simulink model "Sim01_BangBang"  (R2021a)
settings: Solver=FixedStepAuto  StartTime=0.0  StopTime=T  FixedStep=Ts  RelTol=1e-3
values from neighbouring files (symbols this model uses):
  Ts = 1e-3    (= 0.001)    [Sim01_Stability.m]    (also in Sim02_Differentiator.m = 1e-05; Sim03_Differentiator.m = 0.0001)
  umax = 1    [Sim01_Stability.m]    (also in Sim02_Differentiator.m = 20)
  v0 = 0    [Sim01_Stability.m]
  x0 = 0    [Sim01_Stability.m]
undefined symbols (not defined in the file or in its folder): DiscIntNeverNeededParam
settings Model: Creator=XiaoCY  LastModifiedBy=xiaocy
settings SolverCC: AlgebraicLoopSolver=TrustRegion
settings DataIOCC: ReturnWorkspaceOutputs=off
settings DebuggingCC: SFMachineParentedDataDiag=warning

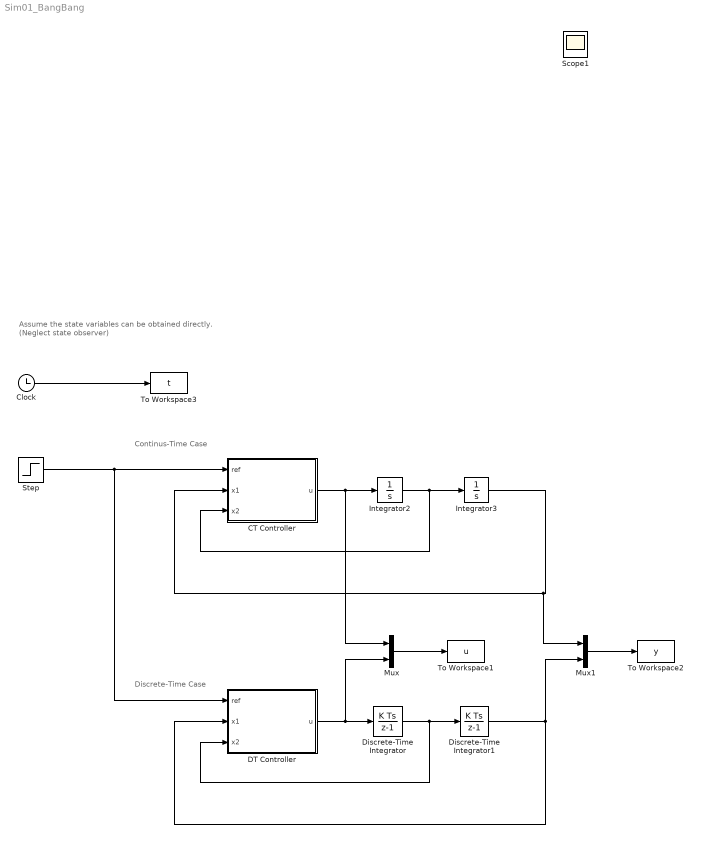
== system Sim01_BangBang ==
  note: Continus-Time Case
  note: Assume the state variables can be obtained directly.
      | (Neglect state observer)
  note: Discrete-Time Case
  CT Controller : Subsystem  VariantControl=dtFlag == 0
  Clock : Clock
  DT Controller : Subsystem  VariantControl=dtFlag == 1
  Discrete-Time Integrator : DiscreteIntegrator  InitialCondition=v0  SampleTime=Ts  ICPrevOutput=DiscIntNeverNeededParam  ICPrevScaledInput=DiscIntNeverNeededParam
  Discrete-Time Integrator1 : DiscreteIntegrator  InitialCondition=x0  SampleTime=Ts  ICPrevOutput=DiscIntNeverNeededParam  ICPrevScaledInput=DiscIntNeverNeededParam
  Integrator2 : Integrator  InitialCondition=v0
  Integrator3 : Integrator  InitialCondition=x0
  Mux : Mux  Inputs=2
  Mux1 : Mux  Inputs=2
  Step : Step  SampleTime=0
  To Workspace1 : ToWorkspace  VariableName=u  SampleTime=Ts
  To Workspace2 : ToWorkspace  VariableName=y  SampleTime=Ts
  To Workspace3 : ToWorkspace  VariableName=t  SampleTime=Ts
  Scope1 : Scope
  wires:
  Clock/1 -> To Workspace3/1
  Integrator2/1 -> CT Controller/3(x2), Integrator3/1
  Integrator3/1 -> Mux1/1, CT Controller/2(x1)
  CT Controller/1(u) -> Mux/1, Integrator2/1
  Step/1 -> DT Controller/1(ref), CT Controller/1(ref)
  DT Controller/1(u) -> Discrete-Time Integrator/1, Mux/2
  Discrete-Time Integrator1/1 -> Mux1/2, DT Controller/2(x1)
  Discrete-Time Integrator/1 -> Discrete-Time Integrator1/1, DT Controller/3(x2)
  Mux/1 -> To Workspace1/1
  Mux1/1 -> To Workspace2/1

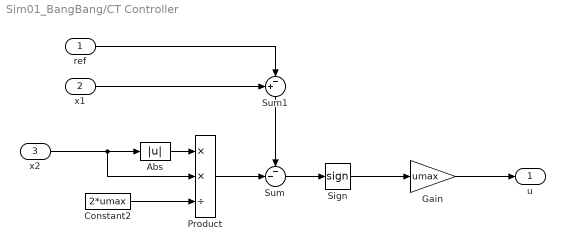
== system Sim01_BangBang/CT Controller ==
  ref : Inport
  x1 : Inport  Port=2
  x2 : Inport  Port=3
  Abs : Abs
  Constant2 : Constant  Value=2*umax
  Gain : Gain  Gain=umax
  Product : Product  Inputs=**/
  Sign : Signum
  Sum : Sum  Inputs=--|
  Sum1 : Sum  Inputs=+-|
  u : Outport
  wires:
  Abs/1 -> Product/1
  Gain/1 -> u/1
  x2/1 -> Product/2, Abs/1
  Constant2/1 -> Product/3
  Sum/1 -> Sign/1
  Sign/1 -> Gain/1
  Product/1 -> Sum/2
  x1/1 -> Sum1/1
  Sum1/1 -> Sum/1
  ref/1 -> Sum1/2

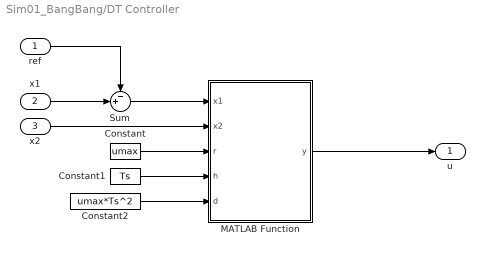
== system Sim01_BangBang/DT Controller ==
  ref : Inport
  x1 : Inport  Port=2
  x2 : Inport  Port=3
  Constant : Constant  Value=umax
  Constant1 : Constant  Value=Ts
  Constant2 : Constant  Value=umax*Ts^2
  MATLAB Function : MATLAB Function  TreatAsAtomicUnit=on  SystemSampleTime=Ts
  Sum : Sum  Inputs=-+|
  u : Outport
  wires:
  x2/1 -> MATLAB Function/2(x2)
  Constant1/1 -> MATLAB Function/4(h)
  Constant/1 -> MATLAB Function/3(r)
  Constant2/1 -> MATLAB Function/5(d)
  x1/1 -> Sum/2
  Sum/1 -> MATLAB Function/1(x1)
  ref/1 -> Sum/1
  MATLAB Function/1(y) -> u/1

== matlab function Sim01_BangBang/DT Controller/MATLAB Function ==
  data: x1 input; y output; x2 input; r input; h input; d input
% Discrete time steepest control synthesis function
% Ref: (ISBN) 978-7-118-05795-9 p.70

%%
function y = fhan(x1,x2,r,h,d)
    fsg = @(x,d) (sign(x+d)-sign(x-d))/2;
    a0 = h*x2;
    y = x1+a0;
    a1 = sqrt(d*(d+8*abs(y)));
    a2 = a0+sign(y)*(a1-d)/2;
    a = (a0+y)*fsg(y,d)+a2*(1-fsg(y,d));
    y = -r*a/d*fsg(a,d)-r*sign(a)*(1-fsg(a,d));
end
